simulink model "system2"  (R2018b)
settings: Solver=VariableStepAuto  StartTime=0.0  StopTime=3  MaxStep=.001  RelTol=1e-3
libraries: cstblocks x4
settings Model: Creator=Abraham Pérez  LastModifiedBy=Abraham Pérez

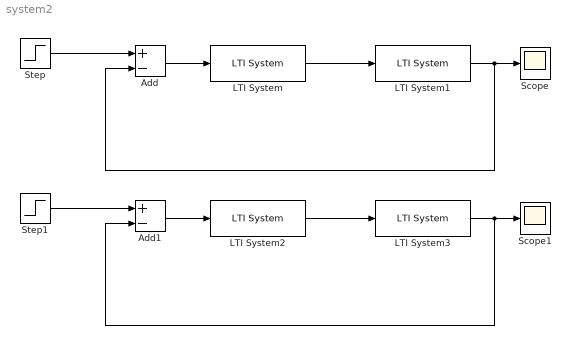
== system system2 ==
  Add : Sum  Inputs=+-
  Add1 : Sum  Inputs=+-
  LTI System : cstblocks/LTI System  sys=C2Lead  IC=[]
  LTI System1 : cstblocks/LTI System  sys=G2  IC=[]
  LTI System2 : cstblocks/LTI System  sys=C2Lag  IC=[]
  LTI System3 : cstblocks/LTI System  sys=G2  IC=[]
  Scope : Scope
  Scope1 : Scope
  Step : Step  Time=0  After=17  SampleTime=0
  Step1 : Step  Time=0  After=9  SampleTime=0
  wires:
  LTI System1/1 -> Add/2, Scope/1
  LTI System/1 -> LTI System1/1
  Add/1 -> LTI System/1
  Step/1 -> Add/1
  Step1/1 -> Add1/1
  LTI System3/1 -> Add1/2, Scope1/1
  Add1/1 -> LTI System2/1
  LTI System2/1 -> LTI System3/1
